simulink model "FM demodulation using PLL"  (R2022b)
settings: Solver=VariableStepAuto  StartTime=0.0  StopTime=1  RelTol=1e-3
libraries: dsparch4 x1, commsynccomp2 x1
settings Model: Creator=mluser  LastModifiedBy=mluser

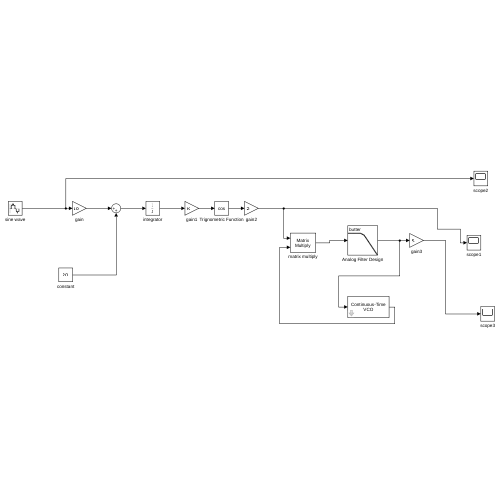
[thumbnail: Simulink's stored preview of the top-level diagram]
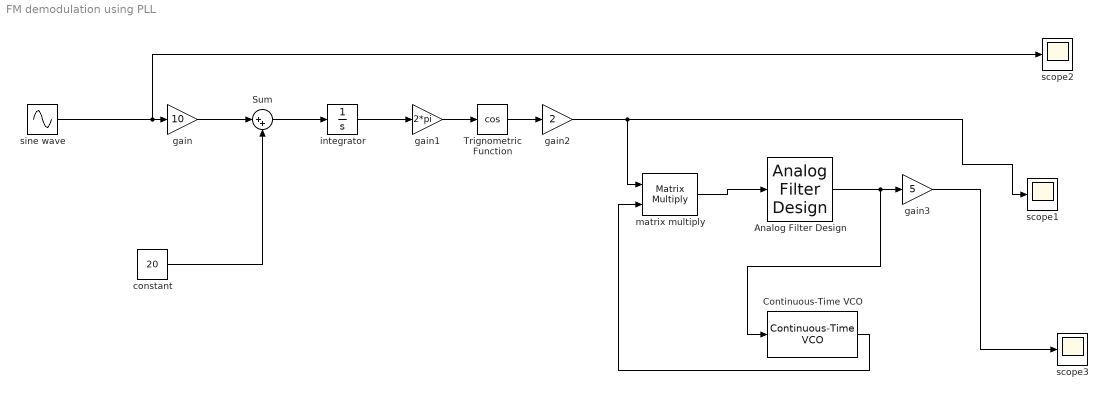
== system FM demodulation using PLL ==
  "Analog Filter Design " : dsparch4/Analog Filter Design  method=Butterworth  filttype=Lowpass  N=3  Wlo=2*pi*2  Whi=80  Rp=2  Rs=40
  Continuous-Time VCO : commsynccomp2/Continuous-Time VCO  Ac=1  Fc=20  Kc=10/(2*pi)  Ph=pi/2
  Sum : Sum  Inputs=|++
  "Trignometric Function " : Trigonometry  Operator=cos
  constant : Constant  Value=20
  gain : Gain  Gain=10
  gain1 : Gain  Gain=2*pi
  gain2 : Gain  Gain=2
  gain3 : Gain  Gain=5
  integrator : Integrator
  matrix multiply : Product  Multiplication=Matrix(*)
  scope1 : Scope
  scope2 : Scope
  scope3 : Scope
  sine wave : Sin  Frequency=2*pi*2  SampleTime=1/1000
  wires:
  gain/1 -> Sum/1
  constant/1 -> Sum/2
  Sum/1 -> integrator/1
  integrator/1 -> gain1/1
  gain1/1 -> "Trignometric Function "/1
  "Trignometric Function "/1 -> gain2/1
  gain2/1 -> scope1/1, matrix multiply/1
  matrix multiply/1 -> "Analog Filter Design "/1
  "Analog Filter Design "/1 -> Continuous-Time VCO/1, gain3/1
  Continuous-Time VCO/1 -> matrix multiply/2
  gain3/1 -> scope3/1
  sine wave/1 -> scope2/1, gain/1
